simulink model "csu_cmv_convert_measured_voltages_collection_hrn"  (R2014b)
settings: Solver=FixedStepDiscrete  StartTime=t0  StopTime=tFinal  FixedStep=sim_dt  RelTol=1e-3
libraries: util_common_lib x1, csu_cmv_convert_measured_voltages_collection_lib x1
settings Model: Creator=escrane  LastModifiedBy=mstewart
settings DebuggingCC: UnderspecifiedInitializationDetection=Classic  MergeDetectMultiDrivingBlocksExec=none  InheritedTsInSrcMsg=none

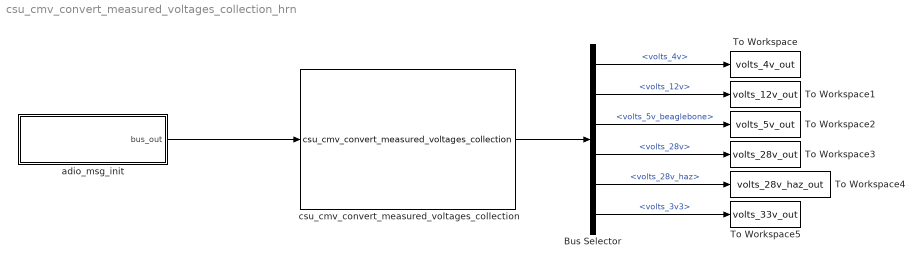
== system csu_cmv_convert_measured_voltages_collection_hrn ==
  Bus Selector : BusSelector  OutputSignals=volts_4v,volts_12v,volts_5v_beaglebone,volts_28v,volts_28v_haz,volts_3v3
  To Workspace : ToWorkspace  VariableName=volts_4v_out  SaveFormat=Timeseries  SampleTime=-1
  To Workspace1 : ToWorkspace  VariableName=volts_12v_out  SaveFormat=Timeseries  SampleTime=-1
  To Workspace2 : ToWorkspace  VariableName=volts_5v_out  SaveFormat=Timeseries  SampleTime=-1
  To Workspace3 : ToWorkspace  VariableName=volts_28v_out  SaveFormat=Timeseries  SampleTime=-1
  To Workspace4 : ToWorkspace  VariableName=volts_28v_haz_out  SaveFormat=Timeseries  SampleTime=-1
  To Workspace5 : ToWorkspace  VariableName=volts_33v_out  SaveFormat=Timeseries  SampleTime=-1
  adio_msg_init : Subsystem
  csu_cmv_convert_measured_voltages_collection : csu_cmv_convert_measured_voltages_collection_lib/csu_cmv_convert_measured_voltages_collection  SystemSampleTime=-1
  wires:
  adio_msg_init/1(bus_out) -> csu_cmv_convert_measured_voltages_collection/1
  csu_cmv_convert_measured_voltages_collection/1 -> Bus Selector/1
  Bus Selector/1 -> To Workspace/1  "<volts_4v>"
  Bus Selector/2 -> To Workspace1/1  "<volts_12v>"
  Bus Selector/3 -> To Workspace2/1  "<volts_5v_beaglebone>"
  Bus Selector/4 -> To Workspace3/1  "<volts_28v>"
  Bus Selector/5 -> To Workspace4/1  "<volts_28v_haz>"
  Bus Selector/6 -> To Workspace5/1  "<volts_3v3>"

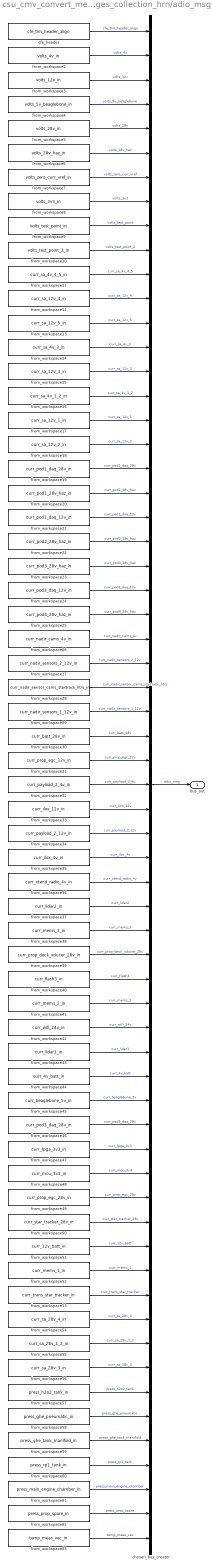
== system csu_cmv_convert_measured_voltages_collection_hrn/adio_msg_init ==
  cfe_header : util_common_lib/cfe_tlm_header_align
  chosen_bus_creator : BusCreator  Inputs=63  OutDataTypeStr=Bus: adio_msg  NonVirtualBus=on
  from_workspace10 : FromWorkspace  VariableName=volts_test_point_2_in
  from_workspace11 : FromWorkspace  VariableName=curr_sa_4v_4_5_in
  from_workspace12 : FromWorkspace  VariableName=curr_sa_12v_4_in
  from_workspace13 : FromWorkspace  VariableName=curr_sa_12v_5_in
  from_workspace14 : FromWorkspace  VariableName=curr_sa_4v_3_in
  from_workspace15 : FromWorkspace  VariableName=curr_sa_12v_3_in
  from_workspace16 : FromWorkspace  VariableName=curr_sa_4v_1_2_in
  from_workspace17 : FromWorkspace  VariableName=curr_sa_12v_1_in
  from_workspace18 : FromWorkspace  VariableName=curr_sa_12v_2_in
  from_workspace19 : FromWorkspace  VariableName=curr_pod1_daq_28v_in
  from_workspace2 : FromWorkspace  VariableName=volts_4v_in
  from_workspace20 : FromWorkspace  VariableName=curr_pod1_28v_haz_in
  from_workspace21 : FromWorkspace  VariableName=curr_pod1_daq_12v_in
  from_workspace22 : FromWorkspace  VariableName=curr_pod2_28v_haz_in
  from_workspace23 : FromWorkspace  VariableName=curr_pod3_28v_haz_in
  from_workspace24 : FromWorkspace  VariableName=curr_pod3_daq_12v_in
  from_workspace25 : FromWorkspace  VariableName=curr_pod4_28v_haz_in
  from_workspace26 : FromWorkspace  VariableName=curr_nadir_cams_4v_in
  from_workspace27 : FromWorkspace  VariableName=curr_nadir_sensors_2_12v_in
  from_workspace28 : FromWorkspace  VariableName=curr_nadir_sensor_cams_startrack_htrs_in
  from_workspace29 : FromWorkspace  VariableName=curr_nadir_sensors_1_12v_in
  from_workspace3 : FromWorkspace  VariableName=volts_12v_in
  from_workspace30 : FromWorkspace  VariableName=curr_batt_28v_in
  from_workspace31 : FromWorkspace  VariableName=curr_prop_egc_12v_in
  from_workspace32 : FromWorkspace  VariableName=curr_payload_2_4v_in
  from_workspace33 : FromWorkspace  VariableName=curr_ilox_12v_in
  from_workspace34 : FromWorkspace  VariableName=curr_payload_2_12v_in
  from_workspace35 : FromWorkspace  VariableName=curr_ilox_4v_in
  from_workspace36 : FromWorkspace  VariableName=curr_xtend_radio_4v_in
  from_workspace37 : FromWorkspace  VariableName=curr_lidar2_in
  from_workspace38 : FromWorkspace  VariableName=curr_mems_3_in
  from_workspace39 : FromWorkspace  VariableName=curr_prop_deck_xducer_28v_in
  from_workspace4 : FromWorkspace  VariableName=volts_5v_beaglebone_in
  from_workspace40 : FromWorkspace  VariableName=curr_flash3_in
  from_workspace41 : FromWorkspace  VariableName=curr_mems_2_in
  from_workspace42 : FromWorkspace  VariableName=curr_wifi_24v_in
  from_workspace43 : FromWorkspace  VariableName=curr_lidar1_in
  from_workspace44 : FromWorkspace  VariableName=curr_4v_batt_in
  from_workspace45 : FromWorkspace  VariableName=curr_beaglebone_5v_in
  from_workspace46 : FromWorkspace  VariableName=curr_pod3_daq_28v_in
  from_workspace47 : FromWorkspace  VariableName=curr_fpga_3v3_in
  from_workspace48 : FromWorkspace  VariableName=curr_mcu_3v3_in
  from_workspace49 : FromWorkspace  VariableName=curr_prop_egc_28v_in
  from_workspace5 : FromWorkspace  VariableName=volts_28v_in
  from_workspace50 : FromWorkspace  VariableName=curr_star_tracker_28v_in
  from_workspace51 : FromWorkspace  VariableName=curr_12v_batt_in
  from_workspace52 : FromWorkspace  VariableName=curr_mems_1_in
  from_workspace53 : FromWorkspace  VariableName=curr_trans_star_tracker_in
  from_workspace54 : FromWorkspace  VariableName=curr_sa_28v_4_in
  from_workspace55 : FromWorkspace  VariableName=curr_sa_28v_1_2_in
  from_workspace56 : FromWorkspace  VariableName=curr_sa_28v_3_in
  from_workspace57 : FromWorkspace  VariableName=press_h2o2_tank_in
  from_workspace58 : FromWorkspace  VariableName=press_ghe_pneumatic_in
  from_workspace59 : FromWorkspace  VariableName=press_ghe_tank_manifold_in
  from_workspace6 : FromWorkspace  VariableName=volts_28v_haz_in
  from_workspace60 : FromWorkspace  VariableName=press_rp1_tank_in
  from_workspace61 : FromWorkspace  VariableName=press_main_engine_chamber_in
  from_workspace62 : FromWorkspace  VariableName=press_prop_spare_in
  from_workspace63 : FromWorkspace  VariableName=temp_meas_vec_in
  from_workspace7 : FromWorkspace  VariableName=volts_zero_curr_vref_in
  from_workspace8 : FromWorkspace  VariableName=volts_3v3_in
  from_workspace9 : FromWorkspace  VariableName=volts_test_point_in
  bus_out : Outport
  wires:
  from_workspace63/1 -> chosen_bus_creator/63  "temp_meas_vec"
  from_workspace62/1 -> chosen_bus_creator/62  "press_prop_spare"
  from_workspace61/1 -> chosen_bus_creator/61  "press_main_engine_chamber"
  from_workspace60/1 -> chosen_bus_creator/60  "press_rp1_tank"
  from_workspace59/1 -> chosen_bus_creator/59  "press_ghe_tank_manifold"
  from_workspace58/1 -> chosen_bus_creator/58  "press_ghe_pneumatic"
  from_workspace57/1 -> chosen_bus_creator/57  "press_h2o2_tank"
  from_workspace56/1 -> chosen_bus_creator/56  "curr_sa_28v_3"
  from_workspace55/1 -> chosen_bus_creator/55  "curr_sa_28v_1_2"
  from_workspace54/1 -> chosen_bus_creator/54  "curr_sa_28v_4"
  from_workspace53/1 -> chosen_bus_creator/53  "curr_trans_star_tracker"
  from_workspace52/1 -> chosen_bus_creator/52  "curr_mems_1"
  from_workspace51/1 -> chosen_bus_creator/51  "curr_12v_batt"
  from_workspace50/1 -> chosen_bus_creator/50  "curr_star_tracker_28v"
  from_workspace49/1 -> chosen_bus_creator/49  "curr_prop_egc_28v"
  from_workspace48/1 -> chosen_bus_creator/48  "curr_mcu_3v3"
  from_workspace47/1 -> chosen_bus_creator/47  "curr_fpga_3v3"
  from_workspace46/1 -> chosen_bus_creator/46  "curr_pod3_daq_28v"
  from_workspace45/1 -> chosen_bus_creator/45  "curr_beaglebone_5v"
  from_workspace44/1 -> chosen_bus_creator/44  "curr_4v_batt"
  from_workspace43/1 -> chosen_bus_creator/43  "curr_lidar1"
  from_workspace42/1 -> chosen_bus_creator/42  "curr_wifi_24v"
  from_workspace41/1 -> chosen_bus_creator/41  "curr_mems_2"
  from_workspace40/1 -> chosen_bus_creator/40  "curr_flash3"
  from_workspace39/1 -> chosen_bus_creator/39  "curr_prop_deck_xducer_28v"
  from_workspace38/1 -> chosen_bus_creator/38  "curr_mems_3"
  from_workspace37/1 -> chosen_bus_creator/37  "curr_lidar2"
  from_workspace36/1 -> chosen_bus_creator/36  "curr_xtend_radio_4v"
  from_workspace35/1 -> chosen_bus_creator/35  "curr_ilox_4v"
  from_workspace34/1 -> chosen_bus_creator/34  "curr_payload_2_12v"
  from_workspace33/1 -> chosen_bus_creator/33  "curr_ilox_12v"
  from_workspace32/1 -> chosen_bus_creator/32  "curr_payload_2_4v"
  from_workspace31/1 -> chosen_bus_creator/31  "curr_prop_egc_12v"
  from_workspace30/1 -> chosen_bus_creator/30  "curr_batt_28v"
  from_workspace29/1 -> chosen_bus_creator/29  "curr_nadir_sensors_1_12v"
  from_workspace28/1 -> chosen_bus_creator/28  "curr_nadir_sensor_cams_startrack_htrs"
  from_workspace27/1 -> chosen_bus_creator/27  "curr_nadir_sensors_2_12v"
  from_workspace26/1 -> chosen_bus_creator/26  "curr_nadir_cams_4v"
  from_workspace25/1 -> chosen_bus_creator/25  "curr_pod4_28v_haz"
  from_workspace24/1 -> chosen_bus_creator/24  "curr_pod3_daq_12v"
  from_workspace23/1 -> chosen_bus_creator/23  "curr_pod3_28v_haz"
  from_workspace22/1 -> chosen_bus_creator/22  "curr_pod2_28v_haz"
  from_workspace21/1 -> chosen_bus_creator/21  "curr_pod1_daq_12v"
  from_workspace20/1 -> chosen_bus_creator/20  "curr_pod1_28v_haz"
  from_workspace19/1 -> chosen_bus_creator/19  "curr_pod1_daq_28v"
  from_workspace18/1 -> chosen_bus_creator/18  "curr_sa_12v_2"
  from_workspace17/1 -> chosen_bus_creator/17  "curr_sa_12v_1"
  from_workspace16/1 -> chosen_bus_creator/16  "curr_sa_4v_1_2"
  from_workspace15/1 -> chosen_bus_creator/15  "curr_sa_12v_3"
  from_workspace14/1 -> chosen_bus_creator/14  "curr_sa_4v_3"
  from_workspace13/1 -> chosen_bus_creator/13  "curr_sa_12v_5"
  from_workspace12/1 -> chosen_bus_creator/12  "curr_sa_12v_4"
  from_workspace11/1 -> chosen_bus_creator/11  "curr_sa_4v_4_5"
  from_workspace10/1 -> chosen_bus_creator/10  "volts_test_point_2"
  from_workspace9/1 -> chosen_bus_creator/9  "volts_test_point"
  from_workspace8/1 -> chosen_bus_creator/8  "volts_3v3"
  from_workspace7/1 -> chosen_bus_creator/7  "volts_zero_curr_vref"
  from_workspace6/1 -> chosen_bus_creator/6  "volts_28v_haz"
  from_workspace5/1 -> chosen_bus_creator/5  "volts_28v"
  from_workspace4/1 -> chosen_bus_creator/4  "volts_5v_beaglebone"
  from_workspace3/1 -> chosen_bus_creator/3  "volts_12v"
  from_workspace2/1 -> chosen_bus_creator/2  "volts_4v"
  cfe_header/1 -> chosen_bus_creator/1  "cfe_tlm_header_align"
  chosen_bus_creator/1 -> bus_out/1  "adio_msg"
